simulink model "skin_temperature_control"  (R2022b)
settings: Solver=ode15s  StartTime=0.0  StopTime=9000  MaxStep=0.4  RelTol=2e-3
undefined symbols (not defined in the file or in its folder): u00, y0
libraries: mpclib x1
settings Model: Creator=Administrator  LastModifiedBy=Administrator
settings DebuggingCC: UnitsInconsistencyMsg=none

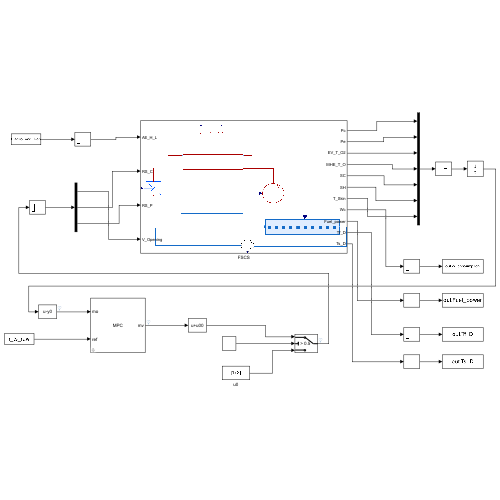
[thumbnail: Simulink's stored preview of the top-level diagram]
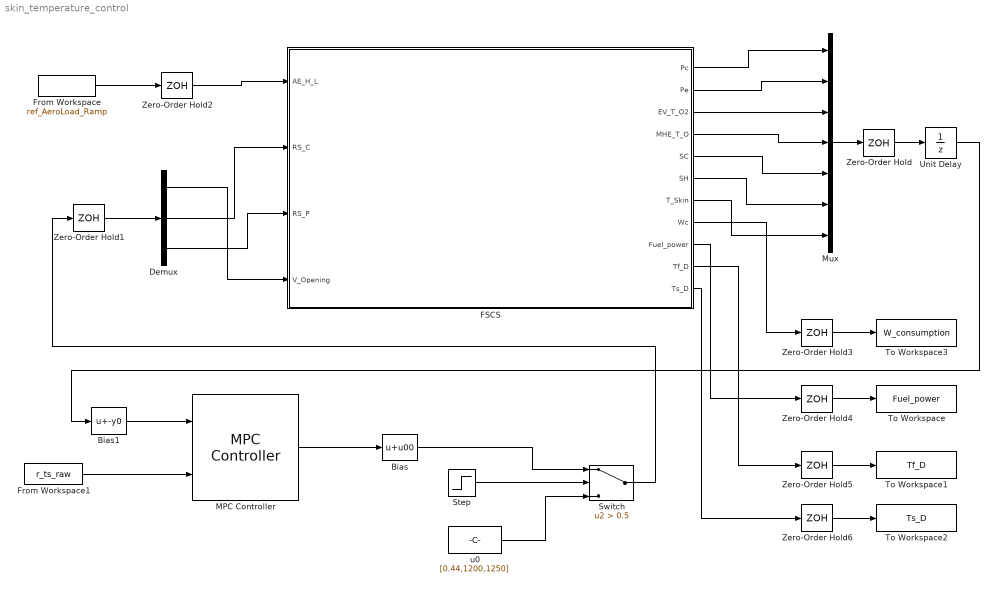
== system skin_temperature_control ==
  Bias : Bias  Bias=u00  SaturateOnIntegerOverflow=off
  Bias1 : Bias  Bias=-y0  SaturateOnIntegerOverflow=off
  Demux : Demux  Outputs=3
  FSCS : Subsystem
      mask Display: image('Skin_Cooling_Systeml.tif'); % Use "Edit Image" on toolstrip to change.
  From Workspace : FromWorkspace  VariableName=ref_AeroLoad_Ramp  SampleTime=2
  From Workspace1 : FromWorkspace  VariableName=r_ts_raw  SampleTime=2
  MPC Controller : mpclib/MPC Controller  SCDEnableBlockLinearizationSpecification=on  mpcobj=mpcobj  is_multiple=0  enable_value=0  return_u0=off  updateMPCinCallerWorkspace=on  md_inport=off  mv_inport=off  uref_inport=off  return_cost=off  return_mvseq=off  return_qpstatus=off  return_xseq=off  return_state=off  return_ovseq=off  state_inport=off  umin_inport=off  umax_inport=off  ymin_inport=off  ymax_inport=off  cc_inport=off  ywt_inport=off  uwt_inport=off  duwt_inport=off  rhoeps_inport=off  pm_inport=off  MaximumP=10  HorizonChoice=FixedHorizon  n_ts=2  n_p=300  n_mv=3  n_md=0  n_ud=1  n_mo=7  n_uo=0  BlockDataType=double  SampleTimeInherited=off  switch_inport=off
  Mux : Mux  Inputs=7
  Step : Step  Time=2000  SampleTime=2
  Switch : Switch  Criteria=u2 > Threshold  Threshold=0.5  SaturateOnIntegerOverflow=off  InputSameDT=off
  To Workspace : ToWorkspace  VariableName=Fuel_power  SaveFormat=Timeseries  SampleTime=-1
  To Workspace1 : ToWorkspace  VariableName=Tf_D  SaveFormat=Timeseries  SampleTime=-1
  To Workspace2 : ToWorkspace  VariableName=Ts_D  SaveFormat=Timeseries  SampleTime=-1
  To Workspace3 : ToWorkspace  VariableName=W_consumption  SaveFormat=Timeseries  SampleTime=-1
  Unit Delay : UnitDelay  SampleTime=2  HasFrameUpgradeWarning=on
  Zero-Order Hold{,1..6} (7 alike) : ZeroOrderHold  SampleTime=2
  u0 : Constant  Value=[0.44,1200,1250]  SampleTime=2
  wires:
  From Workspace1/1 -> MPC Controller/2
  FSCS/1(Pc) -> Mux/1
  FSCS/2(Pe) -> Mux/2
  FSCS/3(EV_T_O2) -> Mux/3
  FSCS/4(MHE_T_O) -> Mux/4
  FSCS/5(SC) -> Mux/5
  FSCS/6(SH) -> Mux/6
  FSCS/7(T_Skin) -> Mux/7
  Demux/1 -> FSCS/4(V_Opening)
  Demux/2 -> FSCS/2(RS_C)
  Demux/3 -> FSCS/3(RS_P)
  Mux/1 -> Zero-Order Hold/1
  Zero-Order Hold/1 -> Unit Delay/1
  Zero-Order Hold2/1 -> FSCS/1(AE_H_L)
  Unit Delay/1 -> Bias1/1
  Bias1/1 -> MPC Controller/1
  Zero-Order Hold1/1 -> Demux/1
  MPC Controller/1 -> Bias/1
  Step/1 -> Switch/2
  Bias/1 -> Switch/1
  u0/1 -> Switch/3
  Switch/1 -> Zero-Order Hold1/1
  From Workspace/1 -> Zero-Order Hold2/1
  Zero-Order Hold6/1 -> To Workspace2/1
  Zero-Order Hold5/1 -> To Workspace1/1
  Zero-Order Hold4/1 -> To Workspace/1
  Zero-Order Hold3/1 -> To Workspace3/1
  FSCS/8(Wc) -> Zero-Order Hold3/1
  FSCS/9(Fuel_power) -> Zero-Order Hold4/1
  FSCS/10(Tf_D) -> Zero-Order Hold5/1
  FSCS/11(Ts_D) -> Zero-Order Hold6/1

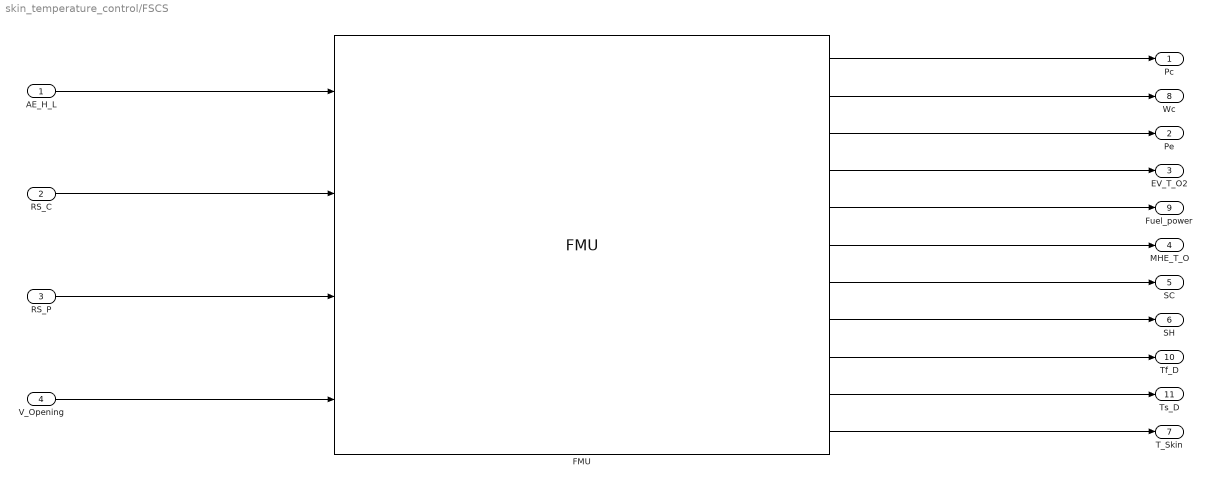
== system skin_temperature_control/FSCS ==
  AE_H_L : Inport
  RS_C : Inport  Port=2
  RS_P : Inport  Port=3
  V_Opening : Inport  Port=4
  FMU : FMU  FMUName=Fuselage_skin_cooling_system.fmu  FMUDebugLogging=on  FMUMode=ModelExchange  compressor=struct('cylinder_volume',4.27069e-4,'cylinder_num',int32(2))  condenser=struct('capacity',880.0,'mass',9.6,'channel_number',int32(14),'panel_number',int32(85))  evaporator=struct('capacity',880.0,'mass',7.84,'channel_number',int32(14),'panel_number',int32(57))  expansion_Valve=struct('flow_area',1.4e-5)  micro_H_E=struct('channel_num',200.0,'fuselage_skin_area',5.0,'mass',40,'wall_capacity',897.0)  pump=struct('Pump_volume',1.5e-4)  compressor_Refrigerant_name=R134a  condenser_Refrigerant_name=R134a  evaporator_Refrigerant_name=R134a  expansion_Valve_Refrigerant_name=R134a  mask(FSCS.System.Fuselage_skin_cooling_system [Model Exchange, v2.0]){}
      settings: MultithreadedSim=off
      mask Display:
      | disp('FSCS.System.Fuselage_skin_cooling_system');
      | port_label('output',1,'Con_pressure');
      | port_label('output',2,'Energy_consumption');
      | port_label('output',3,'Ev_pressure');
      | port_label('output',4,'Ev_tem_o2');
      | port_label('output',5,'Fuel_power');
      | port_label('output',6,'MHE_tem_o');
      | port_label('output',7,'SC');
      | port_label('output',8,'SH');
      | port_label('output',9,'T_micro_f');
      | port_label('output',10,'T_skin');
      | port_label('output',11,'T_skin_av');
      | port_label('input',1,'aerodynamic_heat_load');
      | port_label('input',2,'compressor_rotation_speed');
      | port_label('input',3,'pump_rotation_speed');
      | port_label('input',4,'valve_opening');
  Pc : Outport
  Pe : Outport  Port=2
  EV_T_O2 : Outport  Port=3
  MHE_T_O : Outport  Port=4
  SC : Outport  Port=5
  SH : Outport  Port=6
  T_Skin : Outport  Port=7
  Wc : Outport  Port=8
  Fuel_power : Outport  Port=9
  Tf_D : Outport  Port=10
  Ts_D : Outport  Port=11
  wires:
  AE_H_L/1 -> FMU/1
  RS_C/1 -> FMU/2
  RS_P/1 -> FMU/3
  V_Opening/1 -> FMU/4
  FMU/1 -> Pc/1
  FMU/3 -> Pe/1
  FMU/4 -> EV_T_O2/1
  FMU/6 -> MHE_T_O/1
  FMU/7 -> SC/1
  FMU/8 -> SH/1
  FMU/11 -> T_Skin/1
  FMU/2 -> Wc/1
  FMU/5 -> Fuel_power/1
  FMU/9 -> Tf_D/1
  FMU/10 -> Ts_D/1
